simulink model "controllooppar"  (R2013b)
settings: Solver=ode45  StartTime=0.0  StopTime=300  RelTol=1e-3
model workspace (MAT data in the model file):
  amp = 2225
  freq = 10
  phi = 0.174532925199
libraries: simulink_extras x2
settings Model: Creator=miller.5329  LastModifiedBy=cmiller
settings DataIOCC: LimitDataPoints=off  SignalLoggingSaveFormat=ModelDataLogs
settings OptimizationCC: ExpressionDepthLimit=2147483647
settings DebuggingCC: FcnCallInpInsideContextMsg=EnableAllAsWarning  StateNameClashWarn=warning

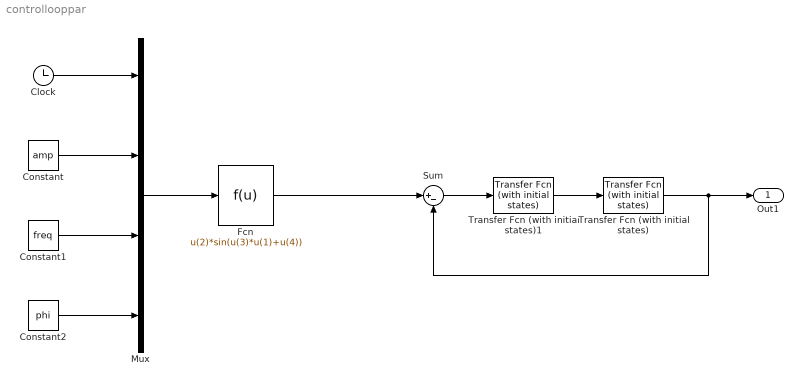
== system controllooppar ==
  Clock : Clock
  Constant : Constant  Value=amp
  Constant1 : Constant  Value=freq
  Constant2 : Constant  Value=phi
  Fcn : Fcn  Expr=u(2)*sin(u(3)*u(1)+u(4))  SampleTime=0
  Mux : Mux
  Sum : Sum  Inputs=|+-
  Transfer Fcn (with initial states) : simulink_extras/Additional Linear/Transfer Fcn (with initial states)  N=[-8*125000 -8*1200 8*1247]  D=[1e6 1e4 20025 100 100]  X0=0
  Transfer Fcn (with initial states)1 : simulink_extras/Additional Linear/Transfer Fcn (with initial states)  N=[1]  D="[50000  1]"  X0=0
  Out1 : Outport
  wires:
  Fcn/1 -> Sum/1
  Sum/1 -> Transfer Fcn (with initial states)1/1
  Transfer Fcn (with initial states)/1 -> Out1/1, Sum/2
  Transfer Fcn (with initial states)1/1 -> Transfer Fcn (with initial states)/1
  Clock/1 -> Mux/1
  Constant/1 -> Mux/2
  Constant1/1 -> Mux/3
  Constant2/1 -> Mux/4
  Mux/1 -> Fcn/1
